simulink model "Demo_CarRealTime2D_cs"  (R2014b)
settings: Solver=ode5  SolverMode=SingleTasking  StartTime=0.0  StopTime=inf  FixedStep=1/1000  RelTol=1e-3
PreLoadFcn:
  | mbxruntime.callbacks.PreLoadFcn(bdroot);
  | check_NUTS_defined;
  | assignin('base',['model_closed_' bdroot],false);
  | addpath('../includes_AEBS');
PostLoadFcn:
  | mbxruntime.callbacks.PostLoadFcn(bdroot);
InitFcn:
  | mbxruntime.callbacks.InitFcn(bdroot);
StartFcn:
  | mbxruntime.callbacks.StartFcn(bdroot);
StopFcn:
  | mbxruntime.callbacks.StopFcn(bdroot);;
  | 
model workspace: external: MAT-File .\Demo_CarRealTime2D_cs_hws.mat (data not in the file)
undefined symbols (not defined in the file or in its folder): Driver_Demands, mbxruntime, tabledata, vicrt_initcallback, vicrt_initmexcallback, vicrt_simulationmanager, warningInitialVelocity, x0
undefined symbols (not defined in the file): Demo_CarRealTime2D_cs_007c1c37f387f47f, Demo_CarRealTime2D_cs_085a64a83ba38cec, Demo_CarRealTime2D_cs_0a7f542d3fc7ab9f, Demo_CarRealTime2D_cs_0d7c72cfaa56dff7, Demo_CarRealTime2D_cs_0de07b35068e3828, Demo_CarRealTime2D_cs_17f4d381375cce95, Demo_CarRealTime2D_cs_1db40a09b08215a9, Demo_CarRealTime2D_cs_2bfa3850c176687b, Demo_CarRealTime2D_cs_35a34f1ba6ce4a22, Demo_CarRealTime2D_cs_378cc77e08d643fb, Demo_CarRealTime2D_cs_409b5c3befba0000, Demo_CarRealTime2D_cs_42628ca5bb62d2f3, Demo_CarRealTime2D_cs_56554a2db408a7f8, Demo_CarRealTime2D_cs_59527455249d7429, Demo_CarRealTime2D_cs_5983ee1b8112afac, Demo_CarRealTime2D_cs_5b5ebcf3ed7bf8e6, Demo_CarRealTime2D_cs_63cbe7fbe16cd5d9, Demo_CarRealTime2D_cs_6e17b9adbf989abf, Demo_CarRealTime2D_cs_6f662a34e5d9a196, Demo_CarRealTime2D_cs_75c4ee8892821e19, Demo_CarRealTime2D_cs_7c64486355814be2, Demo_CarRealTime2D_cs_849809550a2230ef, Demo_CarRealTime2D_cs_87f899bcbe16d8f5, Demo_CarRealTime2D_cs_8e7b50dac25b68a2, Demo_CarRealTime2D_cs_94938e5260f139b3, Demo_CarRealTime2D_cs_983acc940698d1d1, Demo_CarRealTime2D_cs_9d554c72797f76fd, Demo_CarRealTime2D_cs_9d747ee2f15c057f, Demo_CarRealTime2D_cs_ad62a2084d31e898, Demo_CarRealTime2D_cs_b56c8c5f000d30f0, Demo_CarRealTime2D_cs_b95f1b7356e926cc, Demo_CarRealTime2D_cs_BMW_X5_1_Path_pathUniqueID, Demo_CarRealTime2D_cs_BMW_Z3_2_Dynamics_Empty_STATE_BMW_Z3_2_x0, Demo_CarRealTime2D_cs_BMW_Z3_2_Dynamics_Empty_STATE_BMW_Z3_2_y0, Demo_CarRealTime2D_cs_BMW_Z3_2_Dynamics_Empty_STATE_BMW_Z3_2_z0, Demo_CarRealTime2D_cs_BMW_Z3_Path_pathUniqueID, Demo_CarRealTime2D_cs_BMW_Z3_SpeedProfile_speedProfileUniqueID, Demo_CarRealTime2D_cs_c8847ab2e5633224, Demo_CarRealTime2D_cs_c9a0d701286b93fb, Demo_CarRealTime2D_cs_ce758cae7dd1b283, Demo_CarRealTime2D_cs_CrossingPedestrian_Path_pathUniqueID, Demo_CarRealTime2D_cs_CuttingInVehicle_Path_pathUniqueID, Demo_CarRealTime2D_cs_d901ab1c1d2e40bc, Demo_CarRealTime2D_cs_dff70430e5a00a86, Demo_CarRealTime2D_cs_ef038a4f619ad32e, Demo_CarRealTime2D_cs_Female_OverweightAni_1_Path_pathUniqueID, Demo_CarRealTime2D_cs_Ford_Fiesta_1_Path_pathUniqueID, Demo_CarRealTime2D_cs_Ford_FocusWagon_Path_pathUniqueID, Demo_CarRealTime2D_cs_Sphere_1_Dynamics_Empty_STATE_Sphere_1_x0, Demo_CarRealTime2D_cs_Sphere_1_Dynamics_Empty_STATE_Sphere_1_y0, Demo_CarRealTime2D_cs_Sphere_1_Dynamics_Empty_STATE_Sphere_1_z0, WheelL0, WheelL1, WheelR0, WheelR1
libraries: PreScanSimulinkLibrary x15, simulink x15, simulink_extras x15, PreScanUsefulBlocks x2, dspsigops x1
(part 13 of 17)

== system Demo_CarRealTime2D_cs/WheelR1_Ford_FocusWagon/Actuator/visu_Translate ==
  In1 : Inport
  sfun_PositionActuator : S-Function  FunctionName=sfun_PositionActuator  Parameters=SParameter1, SParameter2, SampleTime  EnableBusSupport=off  mask(Legacy Function){SFunctionSpec=void prescan_outputFcn(void ** work1,  PRESCAN_XYZ_DATA u1[1]), SParameter1=uint8([Object3DID 0]), SParameter2=UniqueID, SampleTime=TimeStep, ShowSpec=on}
      mask prompts: SParameter1 "P1:"; SParameter2 "P2:"; SampleTime "Sample time (-1 for inherited):"; ShowSpec "Display function specification"
      mask help:
      | This block allows you to call the legacy functions specified by the following Legacy Code Tool definition:
      | def.SFunctionName = 'sfun_PositionActuator';
      | def.OutputFcnSpec = 'void prescan_outputFcn(void ** work1,  PRESCAN_XYZ_DATA u1[1])';
      | def.StartFcnSpec = 'void prescan_startFcn(void ** work1, uint8 p1[], double p2)';
      | def.TerminateFcnSpec = 'void prescan_terminateFcn(void ** work1)';
      | def.HeaderFiles = {'prescan_positionactuator_data.h', 'prescan_header_data.h', 'prescan_SFunLibrary.h', 'prescan_CreateLogHandler.h', 'prescan_CreateErrorHandler.h'};
      | def.SourceFiles = {'prescan_MexLogHandler.cpp', 'prescan_SimStructErrorHandler.cpp', 'prescan_ConcurrentLogHandler.cpp', 'prescan_ConcurrentErrorHandler.cpp'};
      | def.HostLibFiles = {'sensorinterfaced.lib'};
      | def.TargetLibFiles = {'sensorinterfaced.so'};
      | def.IncPaths = {'.', 'C:\prescandev\vislibrary\vis\..\pimp\include\sensors\InterfaceRTW'};
      | def.SrcPaths = {'.'};
      | def.LibPaths = {'C:\\prescandev\\vislibrary_build\lib'};
      | def.SampleTime = 'parameterized';
      mask Help: <p>This block was generated automatically by the Legacy Code Tool. For detailed help on this tool, call<a href="matlab:legacy_code('help')"> legacy_code('help')</a>.</p>
      mask Callback ShowSpec:
      | if strcmp(get_param(gcbh, 'ShowSpec'), 'on')
      |   set_param(gcbh, 'MaskDisplay', sprintf('fprintf(''%s'');', get_param(gcbh, 'SFunctionSpec')));
      | else
      |   set_param(gcbh, 'MaskDisplay', sprintf('fprintf(''%s'');', get_param(gcbh, 'FunctionName')));
      | end
      mask Display: fprintf('void prescan_outputFcn(void ** work1,  PRESCAN_XYZ_DATA u1[1])');
  wires:
  In1/1 -> sfun_PositionActuator/1

== system Demo_CarRealTime2D_cs/WheelR1_HostVehicle/Actuator/visu_Rotate ==
  In1 : Inport
  sfun_RPYActuator : S-Function  FunctionName=sfun_RPYActuator  Parameters=SParameter1, SParameter2, SampleTime  EnableBusSupport=off  mask(Legacy Function){SFunctionSpec=void prescan_outputFcn(void ** work1,  PRESCAN_XYZ_DATA u1[1]), SParameter1=UniqueID, SParameter2=uint8([Object3DID 0]), SampleTime=TimeStep, ShowSpec=on}
      mask prompts: SParameter1 "P1:"; SParameter2 "P2:"; SampleTime "Sample time (-1 for inherited):"; ShowSpec "Display function specification"
      mask help:
      | This block allows you to call the legacy functions specified by the following Legacy Code Tool definition:
      | def.SFunctionName = 'sfun_PositionActuator';
      | def.OutputFcnSpec = 'void prescan_outputFcn(void ** work1,  PRESCAN_XYZ_DATA u1[1])';
      | def.StartFcnSpec = 'void prescan_startFcn(void ** work1, uint8 p1[], double p2)';
      | def.TerminateFcnSpec = 'void prescan_terminateFcn(void ** work1)';
      | def.HeaderFiles = {'prescan_positionactuator_data.h', 'prescan_header_data.h', 'prescan_SFunLibrary.h', 'prescan_CreateLogHandler.h', 'prescan_CreateErrorHandler.h'};
      | def.SourceFiles = {'prescan_MexLogHandler.cpp', 'prescan_SimStructErrorHandler.cpp', 'prescan_ConcurrentLogHandler.cpp', 'prescan_ConcurrentErrorHandler.cpp'};
      | def.HostLibFiles = {'sensorinterfaced.lib'};
      | def.TargetLibFiles = {'sensorinterfaced.so'};
      | def.IncPaths = {'.', 'C:\prescandev\vislibrary\vis\..\pimp\include\sensors\InterfaceRTW'};
      | def.SrcPaths = {'.'};
      | def.LibPaths = {'C:\\prescandev\\vislibrary_build\lib'};
      | def.SampleTime = 'parameterized';
      mask Help: <p>This block was generated automatically by the Legacy Code Tool. For detailed help on this tool, call<a href="matlab:legacy_code('help')"> legacy_code('help')</a>.</p>
      mask Callback ShowSpec:
      | if strcmp(get_param(gcbh, 'ShowSpec'), 'on')
      |   set_param(gcbh, 'MaskDisplay', sprintf('fprintf(''%s'');', get_param(gcbh, 'SFunctionSpec')));
      | else
      |   set_param(gcbh, 'MaskDisplay', sprintf('fprintf(''%s'');', get_param(gcbh, 'FunctionName')));
      | end
      mask Display: fprintf('void prescan_outputFcn(void ** work1,  PRESCAN_RPY_DATA u1[1])');
  wires:
  In1/1 -> sfun_RPYActuator/1

== system Demo_CarRealTime2D_cs/WheelR1_HostVehicle/Actuator/visu_Translate ==
  In1 : Inport
  sfun_PositionActuator : S-Function  FunctionName=sfun_PositionActuator  Parameters=SParameter1, SParameter2, SampleTime  EnableBusSupport=off  mask(Legacy Function){SFunctionSpec=void prescan_outputFcn(void ** work1,  PRESCAN_XYZ_DATA u1[1]), SParameter1=uint8([Object3DID 0]), SParameter2=UniqueID, SampleTime=TimeStep, ShowSpec=on}
      mask prompts: SParameter1 "P1:"; SParameter2 "P2:"; SampleTime "Sample time (-1 for inherited):"; ShowSpec "Display function specification"
      mask help:
      | This block allows you to call the legacy functions specified by the following Legacy Code Tool definition:
      | def.SFunctionName = 'sfun_PositionActuator';
      | def.OutputFcnSpec = 'void prescan_outputFcn(void ** work1,  PRESCAN_XYZ_DATA u1[1])';
      | def.StartFcnSpec = 'void prescan_startFcn(void ** work1, uint8 p1[], double p2)';
      | def.TerminateFcnSpec = 'void prescan_terminateFcn(void ** work1)';
      | def.HeaderFiles = {'prescan_positionactuator_data.h', 'prescan_header_data.h', 'prescan_SFunLibrary.h', 'prescan_CreateLogHandler.h', 'prescan_CreateErrorHandler.h'};
      | def.SourceFiles = {'prescan_MexLogHandler.cpp', 'prescan_SimStructErrorHandler.cpp', 'prescan_ConcurrentLogHandler.cpp', 'prescan_ConcurrentErrorHandler.cpp'};
      | def.HostLibFiles = {'sensorinterfaced.lib'};
      | def.TargetLibFiles = {'sensorinterfaced.so'};
      | def.IncPaths = {'.', 'C:\prescandev\vislibrary\vis\..\pimp\include\sensors\InterfaceRTW'};
      | def.SrcPaths = {'.'};
      | def.LibPaths = {'C:\\prescandev\\vislibrary_build\lib'};
      | def.SampleTime = 'parameterized';
      mask Help: <p>This block was generated automatically by the Legacy Code Tool. For detailed help on this tool, call<a href="matlab:legacy_code('help')"> legacy_code('help')</a>.</p>
      mask Callback ShowSpec:
      | if strcmp(get_param(gcbh, 'ShowSpec'), 'on')
      |   set_param(gcbh, 'MaskDisplay', sprintf('fprintf(''%s'');', get_param(gcbh, 'SFunctionSpec')));
      | else
      |   set_param(gcbh, 'MaskDisplay', sprintf('fprintf(''%s'');', get_param(gcbh, 'FunctionName')));
      | end
      mask Display: fprintf('void prescan_outputFcn(void ** work1,  PRESCAN_XYZ_DATA u1[1])');
  wires:
  In1/1 -> sfun_PositionActuator/1

== system Demo_CarRealTime2D_cs/Actros_2541_1/SELF_Demux/compas converter/cart2compas ==
  Angle [deg] : Inport
  Constant : Constant  Value=90
  Constant1 : Constant  Value=360
  Gain : Gain  Gain=1/360
  Gain1 : Gain  Gain=360
  Gain2 : Gain  Gain=-1
  Rounding Function : Rounding
  Sum : Sum  Inputs=|-+
  Sum1 : Sum  Inputs=-+|
  Sum2 : Sum  Inputs=++|
  heading [deg] : Outport
  wires:
  Gain/1 -> Rounding Function/1
  Rounding Function/1 -> Gain1/1
  Gain1/1 -> Sum/1
  Angle [deg]/1 -> Sum1/2
  Sum/1 -> Gain2/1
  Sum1/1 -> Gain/1, Sum/2
  Constant/1 -> Sum1/1
  Gain2/1 -> Sum2/2
  Constant1/1 -> Sum2/1
  Sum2/1 -> heading [deg]/1

== system Demo_CarRealTime2D_cs/BMW_X5_1/SELF_Demux/compas converter/cart2compas ==
  Angle [deg] : Inport
  Constant : Constant  Value=90
  Constant1 : Constant  Value=360
  Gain : Gain  Gain=1/360
  Gain1 : Gain  Gain=360
  Gain2 : Gain  Gain=-1
  Rounding Function : Rounding
  Sum : Sum  Inputs=|-+
  Sum1 : Sum  Inputs=-+|
  Sum2 : Sum  Inputs=++|
  heading [deg] : Outport
  wires:
  Gain/1 -> Rounding Function/1
  Rounding Function/1 -> Gain1/1
  Gain1/1 -> Sum/1
  Angle [deg]/1 -> Sum1/2
  Sum/1 -> Gain2/1
  Sum1/1 -> Gain/1, Sum/2
  Constant/1 -> Sum1/1
  Gain2/1 -> Sum2/2
  Constant1/1 -> Sum2/1
  Sum2/1 -> heading [deg]/1

== system Demo_CarRealTime2D_cs/BMW_Z3/SELF_Demux/compas converter/cart2compas ==
  Angle [deg] : Inport
  Constant : Constant  Value=90
  Constant1 : Constant  Value=360
  Gain : Gain  Gain=1/360
  Gain1 : Gain  Gain=360
  Gain2 : Gain  Gain=-1
  Rounding Function : Rounding
  Sum : Sum  Inputs=|-+
  Sum1 : Sum  Inputs=-+|
  Sum2 : Sum  Inputs=++|
  heading [deg] : Outport
  wires:
  Gain/1 -> Rounding Function/1
  Rounding Function/1 -> Gain1/1
  Gain1/1 -> Sum/1
  Angle [deg]/1 -> Sum1/2
  Sum/1 -> Gain2/1
  Sum1/1 -> Gain/1, Sum/2
  Constant/1 -> Sum1/1
  Gain2/1 -> Sum2/2
  Constant1/1 -> Sum2/1
  Sum2/1 -> heading [deg]/1

== system Demo_CarRealTime2D_cs/BMW_Z3_2/SELF_Demux/compas converter/cart2compas ==
  Angle [deg] : Inport
  Constant : Constant  Value=90
  Constant1 : Constant  Value=360
  Gain : Gain  Gain=1/360
  Gain1 : Gain  Gain=360
  Gain2 : Gain  Gain=-1
  Rounding Function : Rounding
  Sum : Sum  Inputs=|-+
  Sum1 : Sum  Inputs=-+|
  Sum2 : Sum  Inputs=++|
  heading [deg] : Outport
  wires:
  Gain/1 -> Rounding Function/1
  Rounding Function/1 -> Gain1/1
  Gain1/1 -> Sum/1
  Angle [deg]/1 -> Sum1/2
  Sum/1 -> Gain2/1
  Sum1/1 -> Gain/1, Sum/2
  Constant/1 -> Sum1/1
  Gain2/1 -> Sum2/2
  Constant1/1 -> Sum2/1
  Sum2/1 -> heading [deg]/1

== system Demo_CarRealTime2D_cs/CrossingPedestrian/SELF_Demux/compas converter/cart2compas ==
  Angle [deg] : Inport
  Constant : Constant  Value=90
  Constant1 : Constant  Value=360
  Gain : Gain  Gain=1/360
  Gain1 : Gain  Gain=360
  Gain2 : Gain  Gain=-1
  Rounding Function : Rounding
  Sum : Sum  Inputs=|-+
  Sum1 : Sum  Inputs=-+|
  Sum2 : Sum  Inputs=++|
  heading [deg] : Outport
  wires:
  Gain/1 -> Rounding Function/1
  Rounding Function/1 -> Gain1/1
  Gain1/1 -> Sum/1
  Angle [deg]/1 -> Sum1/2
  Sum/1 -> Gain2/1
  Sum1/1 -> Gain/1, Sum/2
  Constant/1 -> Sum1/1
  Gain2/1 -> Sum2/2
  Constant1/1 -> Sum2/1
  Sum2/1 -> heading [deg]/1

== system Demo_CarRealTime2D_cs/CuttingInVehicle/SELF_Demux/compas converter/cart2compas ==
  Angle [deg] : Inport
  Constant : Constant  Value=90
  Constant1 : Constant  Value=360
  Gain : Gain  Gain=1/360
  Gain1 : Gain  Gain=360
  Gain2 : Gain  Gain=-1
  Rounding Function : Rounding
  Sum : Sum  Inputs=|-+
  Sum1 : Sum  Inputs=-+|
  Sum2 : Sum  Inputs=++|
  heading [deg] : Outport
  wires:
  Gain/1 -> Rounding Function/1
  Rounding Function/1 -> Gain1/1
  Gain1/1 -> Sum/1
  Angle [deg]/1 -> Sum1/2
  Sum/1 -> Gain2/1
  Sum1/1 -> Gain/1, Sum/2
  Constant/1 -> Sum1/1
  Gain2/1 -> Sum2/2
  Constant1/1 -> Sum2/1
  Sum2/1 -> heading [deg]/1

== system Demo_CarRealTime2D_cs/CuttingInVehicle/Trajectories1/Traj2State1/Traj2State2 ==
  traj : Inport
  MuxState : Subsystem
  Traj2MuxState_Ext : Subsystem
  state : Outport
  wires:
  traj/1 -> Traj2MuxState_Ext/1(Traj)
  MuxState/1(state) -> state/1
  Traj2MuxState_Ext/1(x [m]) -> MuxState/1(x [m])
  Traj2MuxState_Ext/2(y [m]) -> MuxState/2(y [m])
  Traj2MuxState_Ext/3(z [m]) -> MuxState/3(z [m])
  Traj2MuxState_Ext/4(dx [m/s]) -> MuxState/4(dx [m/s])
  Traj2MuxState_Ext/5(dy [m/s]) -> MuxState/5(dy [m/s])
  Traj2MuxState_Ext/6(dz [m/s]) -> MuxState/6(dz [m/s])
  Traj2MuxState_Ext/7(R [rad]) -> MuxState/7(R [rad])
  Traj2MuxState_Ext/8(P [rad]) -> MuxState/8(P [rad])
  Traj2MuxState_Ext/9(Y [rad]) -> MuxState/9(Y [rad])

== system Demo_CarRealTime2D_cs/CuttingInVehicle/Trajectories1/Trajectory_Host_AllSystems/Embeded MATLAB S-Function ==
  gain : Inport
  offset : Inport  Port=2
  MATLAB Function : MATLAB Function  TreatAsAtomicUnit=on  SystemSampleTime=TimeStep
  pos : Outport
  wires:
  offset/1 -> MATLAB Function/2(offset)
  gain/1 -> MATLAB Function/1(gain)
  MATLAB Function/1(y) -> pos/1

== system Demo_CarRealTime2D_cs/Female_OverweightAni_1/SELF_Demux/compas converter/cart2compas ==
  Angle [deg] : Inport
  Constant : Constant  Value=90
  Constant1 : Constant  Value=360
  Gain : Gain  Gain=1/360
  Gain1 : Gain  Gain=360
  Gain2 : Gain  Gain=-1
  Rounding Function : Rounding
  Sum : Sum  Inputs=|-+
  Sum1 : Sum  Inputs=-+|
  Sum2 : Sum  Inputs=++|
  heading [deg] : Outport
  wires:
  Gain/1 -> Rounding Function/1
  Rounding Function/1 -> Gain1/1
  Gain1/1 -> Sum/1
  Angle [deg]/1 -> Sum1/2
  Sum/1 -> Gain2/1
  Sum1/1 -> Gain/1, Sum/2
  Constant/1 -> Sum1/1
  Gain2/1 -> Sum2/2
  Constant1/1 -> Sum2/1
  Sum2/1 -> heading [deg]/1

== system Demo_CarRealTime2D_cs/Ford_Fiesta_1/SELF_Demux/compas converter/cart2compas ==
  Angle [deg] : Inport
  Constant : Constant  Value=90
  Constant1 : Constant  Value=360
  Gain : Gain  Gain=1/360
  Gain1 : Gain  Gain=360
  Gain2 : Gain  Gain=-1
  Rounding Function : Rounding
  Sum : Sum  Inputs=|-+
  Sum1 : Sum  Inputs=-+|
  Sum2 : Sum  Inputs=++|
  heading [deg] : Outport
  wires:
  Gain/1 -> Rounding Function/1
  Rounding Function/1 -> Gain1/1
  Gain1/1 -> Sum/1
  Angle [deg]/1 -> Sum1/2
  Sum/1 -> Gain2/1
  Sum1/1 -> Gain/1, Sum/2
  Constant/1 -> Sum1/1
  Gain2/1 -> Sum2/2
  Constant1/1 -> Sum2/1
  Sum2/1 -> heading [deg]/1

== system Demo_CarRealTime2D_cs/Ford_FocusWagon/SELF_Demux/compas converter/cart2compas ==
  Angle [deg] : Inport
  Constant : Constant  Value=90
  Constant1 : Constant  Value=360
  Gain : Gain  Gain=1/360
  Gain1 : Gain  Gain=360
  Gain2 : Gain  Gain=-1
  Rounding Function : Rounding
  Sum : Sum  Inputs=|-+
  Sum1 : Sum  Inputs=-+|
  Sum2 : Sum  Inputs=++|
  heading [deg] : Outport
  wires:
  Gain/1 -> Rounding Function/1
  Rounding Function/1 -> Gain1/1
  Gain1/1 -> Sum/1
  Angle [deg]/1 -> Sum1/2
  Sum/1 -> Gain2/1
  Sum1/1 -> Gain/1, Sum/2
  Constant/1 -> Sum1/1
  Gain2/1 -> Sum2/2
  Constant1/1 -> Sum2/1
  Sum2/1 -> heading [deg]/1

== system Demo_CarRealTime2D_cs/HostVehicle/Dynamics_UserSpecified/VI-CarRealTime/Input_Bus ==
  Driver_Demands.str_swa : Inport
  Driver_Demands.throttle : Inport  Port=2
  Driver_Demands.brake : Inport  Port=3
  Bus2Map : Subsystem
  Inputs : Subsystem
  VicrtBusAssignment : BusAssignment  AssignedSignals=Driver_Demands.str_swa,Driver_Demands.throttle,Driver_Demands.brake
  vicrt input : Outport
  wires:
  Driver_Demands.brake/1 -> VicrtBusAssignment/4
  Driver_Demands.throttle/1 -> VicrtBusAssignment/3
  Driver_Demands.str_swa/1 -> VicrtBusAssignment/2
  Inputs/1(Inputs) -> VicrtBusAssignment/1  "Inputs"
  VicrtBusAssignment/1 -> Bus2Map/1(Bus In)
  Bus2Map/1(Map Out) -> vicrt input/1

== system Demo_CarRealTime2D_cs/HostVehicle/Dynamics_UserSpecified/VI-CarRealTime/Output_Bus ==
  Outputs : Inport
  IOmap2bus : Subsystem
  VicrtBusSelector : BusSelector  InitFcn=warning('off','Simulink:blocks:BusSelectorDuplicateLeafSignalInMuxedOutput');  StartFcn=warning('on','Simulink:blocks:BusSelectorDuplicateLeafSignalInMuxedOutput');  OutputSignals=ges_chassis_XFORM.X,ges_chassis_XFORM.Y,ges_chassis_XFORM.Z,Vehicle.CM_Body_Fixed_Vx,Vehicle.CM_Body_Fixed_Vy,Vehicle.CM_Body_Fixed_Vz,Vehicle.Euler_Roll,Vehicle.Pitch,Vehicle.Yaw,Wheel.wheel_center_dispz.front_left,Wheel.wheel_center_dispz.front_right,Wheel.wheel_center_dispz.rear_left,Wheel.wheel_center_dispz.rear_right,engine.engine_rpm,Vehicle.CM_Body_Fixed_Ax
  ges_chassis_XFORM.X : Outport
  ges_chassis_XFORM.Y : Outport  Port=2
  ges_chassis_XFORM.Z : Outport  Port=3
  Vehicle.CM_Body_Fixed_Vx : Outport  Port=4
  Vehicle.CM_Body_Fixed_Vy : Outport  Port=5
  Vehicle.CM_Body_Fixed_Vz : Outport  Port=6
  Vehicle.Euler_Roll : Outport  Port=7
  Vehicle.Pitch : Outport  Port=8
  Vehicle.Yaw : Outport  Port=9
  Wheel.wheel_center_dispz.front_left : Outport  Port=10
  Wheel.wheel_center_dispz.front_right : Outport  Port=11
  Wheel.wheel_center_dispz.rear_left : Outport  Port=12
  Wheel.wheel_center_dispz.rear_right : Outport  Port=13
  engine.engine_rpm : Outport  Port=14
  Vehicle.CM_Body_Fixed_Ax : Outport  Port=15
  wires:
  VicrtBusSelector/15 -> Vehicle.CM_Body_Fixed_Ax/1  "<CM_Body_Fixed_Ax>"
  VicrtBusSelector/14 -> engine.engine_rpm/1  "<engine_rpm>"
  VicrtBusSelector/13 -> Wheel.wheel_center_dispz.rear_right/1  "<rear_right>"
  VicrtBusSelector/12 -> Wheel.wheel_center_dispz.rear_left/1  "<rear_left>"
  VicrtBusSelector/11 -> Wheel.wheel_center_dispz.front_right/1  "<front_right>"
  VicrtBusSelector/10 -> Wheel.wheel_center_dispz.front_left/1  "<front_left>"
  VicrtBusSelector/9 -> Vehicle.Yaw/1  "<Yaw>"
  VicrtBusSelector/8 -> Vehicle.Pitch/1  "<Pitch>"
  VicrtBusSelector/7 -> Vehicle.Euler_Roll/1  "<Euler_Roll>"
  VicrtBusSelector/6 -> Vehicle.CM_Body_Fixed_Vz/1  "<CM_Body_Fixed_Vz>"
  VicrtBusSelector/5 -> Vehicle.CM_Body_Fixed_Vy/1  "<CM_Body_Fixed_Vy>"
  VicrtBusSelector/4 -> Vehicle.CM_Body_Fixed_Vx/1  "<CM_Body_Fixed_Vx>"
  VicrtBusSelector/3 -> ges_chassis_XFORM.Z/1  "<Z>"
  VicrtBusSelector/2 -> ges_chassis_XFORM.Y/1  "<Y>"
  VicrtBusSelector/1 -> ges_chassis_XFORM.X/1  "<X>"
  Outputs/1 -> IOmap2bus/1(In)
  IOmap2bus/1(Out) -> VicrtBusSelector/1

== system Demo_CarRealTime2D_cs/HostVehicle/Dynamics_UserSpecified/VI-CarRealTime/vicrt_mex Standard ==
  In1 : Inport
  vicrt_mex : S-Function  InitFcn=vicrt_initmexcallback(gcb);  FunctionName=vicrt_mex  Parameters=vicrt_inputfile,vicrt_outprefix,AniFlag,intStep,inpPortDim,outPortDim  EnableBusSupport=off
  Out1 : Outport
  wires:
  In1/1 -> vicrt_mex/1
  vicrt_mex/1 -> Out1/1

== system Demo_CarRealTime2D_cs/HostVehicle/PathFollower_Preview_1/LateralController/Calculate delta steering error ==
  In1 : Inport
  In2 : Inport  Port=2
  In3 : Inport  Port=3
  In4 : Inport  Port=4
  In5 : Inport  Port=5
  In6 : Inport  Port=6
  In7 : Inport  Port=7
  In8 : Inport  Port=8
  In9 : Inport  Port=9
  In10 : Inport  Port=10
  In11 : Inport  Port=11
  In12 : Inport  Port=12
  eml_delta_steering_error : MATLAB Function  TreatAsAtomicUnit=on  RTWFcnName=sfun_delta_steering_error  RTWFileName=sfun_delta_steering_error
      settings: RTWFileNameOpts=User specified
  Out1 : Outport
  wires:
  In3/1 -> eml_delta_steering_error/3(t_Preview_LatCtrl)
  In2/1 -> eml_delta_steering_error/2(v_x_vehicle_Min)
  In12/1 -> eml_delta_steering_error/12(wheelbase)
  In11/1 -> eml_delta_steering_error/11(Pos_x_CoG_Vehicle)
  In10/1 -> eml_delta_steering_error/10(e_Lat)
  In9/1 -> eml_delta_steering_error/9(inertia_z_vehicle_total)
  In8/1 -> eml_delta_steering_error/8(m_vehicle_total)
  eml_delta_steering_error/1(delta_steeringwheeltotal) -> Out1/1
  In7/1 -> eml_delta_steering_error/7(CorneringStiffness_Tyres_Rear)
  In6/1 -> eml_delta_steering_error/6(CorneringStiffness_Tyres_Front)
  In5/1 -> eml_delta_steering_error/5(yawrate_vehicle)
  In4/1 -> eml_delta_steering_error/4(v_y_vehicle)
  In1/1 -> eml_delta_steering_error/1(v_x_vehicle)

== system Demo_CarRealTime2D_cs/HostVehicle/PathFollower_Preview_1/LateralController/SteeringWheelAngle ==
  Angle_Steering[rad] : Inport
  i_Steering[] : Inport  Port=2
  Angle_SteeringWheel_Last[deg] : Inport  Port=3
  LatCtrl1_Enable[0Off|1On] : Inport  Port=4
  Angle_Max_SteeringWheel[deg]1 : Constant  Value=Angle_Max_SteeringWheel  SampleTime=CSSampleTime
  Const_t_PT1_LatCtrl[s] : Constant  Value=DelayTime  SampleTime=CSSampleTime
  FirstOrderDynamics : Subsystem  mask(First Order Dynamics){}
      mask Display:
      | port_label('input',1,'In')
      | port_label('input',2,'T')
      | port_label('input',3,'Reset')
      | port_label('input',4,'x0')
      | 
      | plot([0.4 0.95], [0.1 0.1]);
      | plot([0.4 0.4], [0.1 0.95]);
      | plot(0.4 + 0.5*[0:0.1:1],0.8- 0.7 * exp(-5*[0:0.1:1]));
  Gain : Gain  SaturateOnIntegerOverflow=on  OutDataTypeStr=Inherit: Same as input  ParamDataTypeStr=Inherit: Same as input
  Product : Product  SaturateOnIntegerOverflow=on  OutDataTypeStr=Inherit: Same as first input
  Rate Limiter : RateLimiter  RisingSlewLimit=MaxSteeringRate  FallingSlewLimit=-MaxSteeringRate  SampleTimeMode=inherited
  Sat_Total : Subsystem
      mask Display:
      | plot([0.25 0.4 0.6 0.75],[0.2 0.2 0.8 0.8])
      | port_label('input',2,'Lim')
      | port_label('output',2,'Info')
  Terminator1 : Terminator
  rad2deg : Gain  Gain=180/pi  SaturateOnIntegerOverflow=on  OutDataTypeStr=Inherit: Same as input  ParamDataTypeStr=Inherit: Same as input
  Angle_SteeringWheel[deg] : Outport
  wires:
  Rate Limiter/1 -> FirstOrderDynamics/1(In)
  Gain/1 -> FirstOrderDynamics/3(Reset)
  Angle_SteeringWheel_Last[deg]/1 -> FirstOrderDynamics/4(x0)
  LatCtrl1_Enable[0Off|1On]/1 -> Gain/1
  Const_t_PT1_LatCtrl[s]/1 -> FirstOrderDynamics/2(TimeConstant[s])
  Sat_Total/2(Sat_Info) -> Terminator1/1
  Angle_Steering[rad]/1 -> rad2deg/1
  i_Steering[]/1 -> Product/2
  rad2deg/1 -> Product/1
  Product/1 -> Sat_Total/1(In)
  Sat_Total/1(Sat_Total) -> Rate Limiter/1
  FirstOrderDynamics/1(Out) -> Angle_SteeringWheel[deg]/1
  Angle_Max_SteeringWheel[deg]1/1 -> Sat_Total/2(Sat_Limit)

== system Demo_CarRealTime2D_cs/HostVehicle/PathFollower_Preview_1/LateralController/s_Preview_LatCtrl ==
  v_x_Vehicle[m|s] : Inport
  v_x_Vehicle_Min[m|s] : Inport  Port=2
  t_Preview_LatCtrl[s] : Inport  Port=3
  Max : MinMax  Function=max  Inputs=2  SaturateOnIntegerOverflow=on  InputSameDT=on
  Prod_s_Min : Product  SaturateOnIntegerOverflow=on  OutDataTypeStr=Inherit: Same as first input
  Product : Product  SaturateOnIntegerOverflow=on  OutDataTypeStr=Inherit: Same as first input
  s_Preview_LatCtrl[m] : Outport
  wires:
  Max/1 -> s_Preview_LatCtrl[m]/1
  Prod_s_Min/1 -> Max/2
  v_x_Vehicle_Min[m|s]/1 -> Prod_s_Min/2
  t_Preview_LatCtrl[s]/1 -> Prod_s_Min/1, Product/2
  Product/1 -> Max/1
  v_x_Vehicle[m|s]/1 -> Product/1

== system Demo_CarRealTime2D_cs/HostVehicle/PathFollower_Preview_1/LongitudinalController/Check_Initial_Velocity ==
  " v_actual_[m|s]" : Inport
  Initial_Velocity_[m|s] : Inport  Port=2
  > eps : simulink/Logic and Bit Operations/Compare To Constant  relop=>  const=0.1  OutDataTypeStr=boolean
  Abs : Abs
  Assertion : Assertion  AssertionFailFcn=warningInitialVelocity(PathFollowerBlockPath);  StopWhenAssertionFail=off
  Constant : Constant  Value=false
  First ? : Memory  X0=1
  Logical Operator : Logic  AllPortsSameDT=off  OutDataTypeStr=boolean
  Logical Operator1 : Logic  Operator=NOT  AllPortsSameDT=off  OutDataTypeStr=boolean
  Sum : Sum  Inputs=+-
  wires:
  Logical Operator1/1 -> Assertion/1
  Logical Operator/1 -> Logical Operator1/1
  Constant/1 -> First ?/1
  First ?/1 -> Logical Operator/2
  > eps/1 -> Logical Operator/1
  Sum/1 -> Abs/1
  Abs/1 -> > eps/1
  Initial_Velocity_[m|s]/1 -> Sum/2
  " v_actual_[m|s]"/1 -> Sum/1

== system Demo_CarRealTime2D_cs/HostVehicle/PathFollower_Preview_1/LongitudinalController/If Desired Velocity = 0 ==
  In1 : Inport
  Action Port : ActionPort  InitializeStates=reset  PropagateVarSize=During execution
  constant : Constant  Value=0
  constant1 : Constant  Value=150
  throttle [%] : Outport  InitialOutput=[0]
  brake pressure [bar] : Outport  Port=2  InitialOutput=[150]
  Auto_GearShift : Outport  Port=3
  wires:
  In1/1 -> Auto_GearShift/1
  constant/1 -> throttle [%]/1
  constant1/1 -> brake pressure [bar]/1

== system Demo_CarRealTime2D_cs/HostVehicle/PathFollower_Preview_1/LongitudinalController/If Desired Velocity ~= 0 ==
  note: No brake/throttle actions
      | in case of small ctrl error,
      |  in order to prevent nervous
      | ctrl behaviour
  note: CONSTANT VELOCITY CONTROL
  In1 : Inport
  Desired Velocity [m/s] : Inport  Port=2
  Action Port : ActionPort  InitializeStates=reset  PropagateVarSize=During execution
  Dead Zone1 : DeadZone  LowerValue=-10  UpperValue=1  SaturateOnIntegerOverflow=on
  Gain1 : Gain  Gain=-1
  Gain2 : Gain  Gain=1.5
  Limiter_brake : Saturate  UpperLimit=150  LowerLimit=0
  Limiter_throttle : Saturate  UpperLimit=100  LowerLimit=0
  PID_AWU : Subsystem  mask(PID Controller){P=LongCtrl_P, I=LongCtrl_I, D=LongCtrl_D}
      mask prompts: P "Proportional:"; I "Integral:"; D "Derivative:"
      mask help:
      | Enter expressions for proportional, integral, and derivative terms.
      | P+I/s+Ds
      mask Help: This block implements a PID controller where parameters are entered for the Proportional, Integral and Derivative terms. Unmask this block to see how it works. The derivative term is implemented using a true derivative block.
      mask Display: disp('PID')
  throttle [%] : Outport
  brake pressure [bar] : Outport  Port=2
  Auto_GearShift : Outport  Port=3
  wires:
  Dead Zone1/1 -> Gain2/1, Limiter_throttle/1
  Gain1/1 -> Limiter_brake/1
  Gain2/1 -> Gain1/1
  PID_AWU/1(u) -> Dead Zone1/1
  Desired Velocity [m/s]/1 -> PID_AWU/1(e)
  In1/1 -> Auto_GearShift/1
  Limiter_brake/1 -> brake pressure [bar]/1
  Limiter_throttle/1 -> throttle [%]/1  "throttle"

== system Demo_CarRealTime2D_cs/HostVehicle/PathFollower_Preview_1/LongitudinalController/Memory External IC ==
  note: Xnew
  note: Initial Value
  u : Inport
  IC : Inport  Port=2
  FixPt Constant : Constant  DisableCoverage=on  Value=0  OutDataTypeStr=fixdt(0,8,0)
  FixPt Data Type Duplicate1 : DataTypeDuplicate  DisableCoverage=on  NumInputPorts=3
  Init : Switch  Criteria=u2 ~= 0  OutDataTypeStr=Inherit: Inherit via back propagation  ZeroCross=off
  Memory : Memory  X0=1  InheritSampleTime=on
  Memory1 : Memory  InheritSampleTime=on
  y : Outport
  wires:
  Memory1/1 -> Init/3  "Xold"
  Init/1 -> y/1, FixPt Data Type Duplicate1/1
  Memory/1 -> Init/2
  FixPt Constant/1 -> Memory/1
  u/1 -> Memory1/1, FixPt Data Type Duplicate1/2
  IC/1 -> Init/1, FixPt Data Type Duplicate1/3

== system Demo_CarRealTime2D_cs/HostVehicle/SELF_Demux/compas converter/cart2compas ==
  Angle [deg] : Inport
  Constant : Constant  Value=90
  Constant1 : Constant  Value=360
  Gain : Gain  Gain=1/360
  Gain1 : Gain  Gain=360
  Gain2 : Gain  Gain=-1
  Rounding Function : Rounding
  Sum : Sum  Inputs=|-+
  Sum1 : Sum  Inputs=-+|
  Sum2 : Sum  Inputs=++|
  heading [deg] : Outport
  wires:
  Gain/1 -> Rounding Function/1
  Rounding Function/1 -> Gain1/1
  Gain1/1 -> Sum/1
  Angle [deg]/1 -> Sum1/2
  Sum/1 -> Gain2/1
  Sum1/1 -> Gain/1, Sum/2
  Constant/1 -> Sum1/1
  Gain2/1 -> Sum2/2
  Constant1/1 -> Sum2/1
  Sum2/1 -> heading [deg]/1

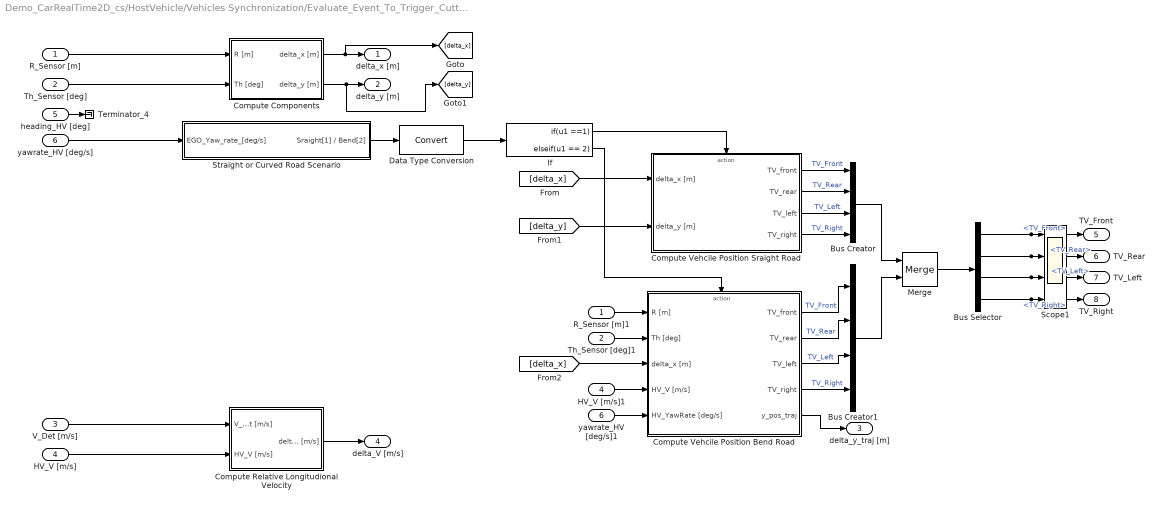
== system Demo_CarRealTime2D_cs/HostVehicle/Vehicles Synchronization/Evaluate_Event_To_Trigger_CuttingVehicle/Evaluate Experiment Conditions  ==
  R_Sensor [m] : Inport
  Th_Sensor [deg] : Inport  Port=2
  V_Det [m/s] : Inport  Port=3
  HV_V [m/s] : Inport  Port=4
  heading_HV [deg] : Inport  Port=5
  yawrate_HV [deg/s] : Inport  Port=6
  Bus Creator : BusCreator
  Bus Creator1 : BusCreator
  Bus Selector : BusSelector  OutputSignals=TV_Front,TV_Rear,TV_Left,TV_Right
  Compute Components : Subsystem
  Compute Relative Longitudional Velocity : Subsystem
  Compute Vehcile Position Bend Road : Subsystem  TreatAsAtomicUnit=on
  Compute Vehcile Position Sraight Road : Subsystem  TreatAsAtomicUnit=on
  Data Type Conversion : DataTypeConversion
  HV_V [m/s]1 : InportShadow  Port=4
  If : If  IfExpression=u1 ==1  ElseIfExpressions=u1 == 2  ShowElse=off
  Merge : Merge
  R_Sensor [m]1 : InportShadow
  Scope1 : Scope  NumInputPorts=4
      settings: YMin=1~0~0~0.95  YMax=2~1~1~1.05
  Straight or Curved Road Scenario : Subsystem
  Terminator_4 : Terminator
  Th_Sensor [deg]1 : InportShadow  Port=2
  yawrate_HV [deg/s]1 : InportShadow  Port=6
  delta_x [m] : Outport
  delta_y [m] : Outport  Port=2
  delta_y_traj [m] : Outport  Port=3
  delta_V [m/s] : Outport  Port=4
  TV_Front : Outport  Port=5
  TV_Rear : Outport  Port=6
  TV_Left : Outport  Port=7
  TV_Right : Outport  Port=8
  wires:
  Bus Selector/4 -> TV_Right/1, Scope1/4  "<TV_Right>"
  Bus Selector/3 -> TV_Left/1, Scope1/3  "<TV_Left>"
  Bus Selector/2 -> TV_Rear/1, Scope1/2  "<TV_Rear>"
  Bus Selector/1 -> TV_Front/1, Scope1/1  "<TV_Front>"
  Compute Vehcile Position Bend Road/5(y_pos_traj) -> delta_y_traj [m]/1
  heading_HV [deg]/1 -> Terminator_4/1
  Merge/1 -> Bus Selector/1
  Bus Creator1/1 -> Merge/2
  Bus Creator/1 -> Merge/1
  Compute Vehcile Position Bend Road/4(TV_right) -> Bus Creator1/4  "TV_Right"
  Compute Vehcile Position Bend Road/3(TV_left) -> Bus Creator1/3  "TV_Left"
  Compute Vehcile Position Bend Road/2(TV_rear) -> Bus Creator1/2  "TV_Rear"
  Compute Vehcile Position Bend Road/1("TV_front ") -> Bus Creator1/1  "TV_Front"
  Compute Vehcile Position Sraight Road/2(TV_rear) -> Bus Creator/2  "TV_Rear"
  Compute Vehcile Position Sraight Road/3(TV_left) -> Bus Creator/3  "TV_Left"
  Compute Vehcile Position Sraight Road/1("TV_front ") -> Bus Creator/1  "TV_Front"
  Compute Vehcile Position Sraight Road/4(TV_right) -> Bus Creator/4  "TV_Right"
  yawrate_HV [deg/s]1/1 -> Compute Vehcile Position Bend Road/5(HV_YawRate [deg/s])
  HV_V [m/s]1/1 -> Compute Vehcile Position Bend Road/4(HV_V [m/s])
  [delta_x] -> Compute Vehcile Position Bend Road/3(delta_x [m])
  [delta_y] -> Compute Vehcile Position Sraight Road/2(delta_y [m])
  [delta_x] -> Compute Vehcile Position Sraight Road/1(delta_x [m])
  Th_Sensor [deg]1/1 -> Compute Vehcile Position Bend Road/2(Th [deg])
  R_Sensor [m]1/1 -> Compute Vehcile Position Bend Road/1(R [m])
  If/2 -> Compute Vehcile Position Bend Road/Action
  If/1 -> Compute Vehcile Position Sraight Road/Action
  Data Type Conversion/1 -> If/1
  Straight or Curved Road Scenario/1(Sraight[1] / Bend[2]) -> Data Type Conversion/1
  yawrate_HV [deg/s]/1 -> Straight or Curved Road Scenario/1(EGO_Yaw_rate_[deg/s])
  Th_Sensor [deg]/1 -> Compute Components/2(Th [deg])
  Compute Relative Longitudional Velocity/1(delta_V [m/s]) -> delta_V [m/s]/1
  HV_V [m/s]/1 -> Compute Relative Longitudional Velocity/2(HV_V [m/s])
  V_Det [m/s]/1 -> Compute Relative Longitudional Velocity/1(V_Det [m/s])
  Compute Components/2(delta_y [m]) -> [delta_y], delta_y [m]/1
  Compute Components/1(delta_x [m]) -> [delta_x], delta_x [m]/1
  R_Sensor [m]/1 -> Compute Components/1(R [m])

== system Demo_CarRealTime2D_cs/Male_Regular_LeaningBack_2/SELF_Demux/compas converter/cart2compas ==
  Angle [deg] : Inport
  Constant : Constant  Value=90
  Constant1 : Constant  Value=360
  Gain : Gain  Gain=1/360
  Gain1 : Gain  Gain=360
  Gain2 : Gain  Gain=-1
  Rounding Function : Rounding
  Sum : Sum  Inputs=|-+
  Sum1 : Sum  Inputs=-+|
  Sum2 : Sum  Inputs=++|
  heading [deg] : Outport
  wires:
  Gain/1 -> Rounding Function/1
  Rounding Function/1 -> Gain1/1
  Gain1/1 -> Sum/1
  Angle [deg]/1 -> Sum1/2
  Sum/1 -> Gain2/1
  Sum1/1 -> Gain/1, Sum/2
  Constant/1 -> Sum1/1
  Gain2/1 -> Sum2/2
  Constant1/1 -> Sum2/1
  Sum2/1 -> heading [deg]/1

== system Demo_CarRealTime2D_cs/Sphere_1/SELF_Demux/compas converter/cart2compas ==
  Angle [deg] : Inport
  Constant : Constant  Value=90
  Constant1 : Constant  Value=360
  Gain : Gain  Gain=1/360
  Gain1 : Gain  Gain=360
  Gain2 : Gain  Gain=-1
  Rounding Function : Rounding
  Sum : Sum  Inputs=|-+
  Sum1 : Sum  Inputs=-+|
  Sum2 : Sum  Inputs=++|
  heading [deg] : Outport
  wires:
  Gain/1 -> Rounding Function/1
  Rounding Function/1 -> Gain1/1
  Gain1/1 -> Sum/1
  Angle [deg]/1 -> Sum1/2
  Sum/1 -> Gain2/1
  Sum1/1 -> Gain/1, Sum/2
  Constant/1 -> Sum1/1
  Gain2/1 -> Sum2/2
  Constant1/1 -> Sum2/1
  Sum2/1 -> heading [deg]/1

== system Demo_CarRealTime2D_cs/Toyota_Previa_1/SELF_Demux/compas converter/cart2compas ==
  Angle [deg] : Inport
  Constant : Constant  Value=90
  Constant1 : Constant  Value=360
  Gain : Gain  Gain=1/360
  Gain1 : Gain  Gain=360
  Gain2 : Gain  Gain=-1
  Rounding Function : Rounding
  Sum : Sum  Inputs=|-+
  Sum1 : Sum  Inputs=-+|
  Sum2 : Sum  Inputs=++|
  heading [deg] : Outport
  wires:
  Gain/1 -> Rounding Function/1
  Rounding Function/1 -> Gain1/1
  Gain1/1 -> Sum/1
  Angle [deg]/1 -> Sum1/2
  Sum/1 -> Gain2/1
  Sum1/1 -> Gain/1, Sum/2
  Constant/1 -> Sum1/1
  Gain2/1 -> Sum2/2
  Constant1/1 -> Sum2/1
  Sum2/1 -> heading [deg]/1

== system Demo_CarRealTime2D_cs/CuttingInVehicle/Trajectories1/Traj2State1/Traj2State2/MuxState ==
  x [m] : Inport
  y [m] : Inport  Port=2
  z [m] : Inport  Port=3
  dx [m/s] : Inport  Port=4
  dy [m/s] : Inport  Port=5
  dz [m/s] : Inport  Port=6
  R [rad] : Inport  Port=7
  P [rad] : Inport  Port=8
  Y [rad] : Inport  Port=9
  Mux : Mux  Inputs=9
  state : Outport
  wires:
  Mux/1 -> state/1
  dx [m/s]/1 -> Mux/4
  dy [m/s]/1 -> Mux/5
  dz [m/s]/1 -> Mux/6
  R [rad]/1 -> Mux/7
  P [rad]/1 -> Mux/8
  Y [rad]/1 -> Mux/9
  x [m]/1 -> Mux/1
  y [m]/1 -> Mux/2
  z [m]/1 -> Mux/3

== system Demo_CarRealTime2D_cs/CuttingInVehicle/Trajectories1/Traj2State1/Traj2State2/Traj2MuxState_Ext ==
  Traj : Inport
  Terminator{1..9} (9 alike) : Terminator
  demux : Subsystem
  x [m] : Outport
  y [m] : Outport  Port=2
  z [m] : Outport  Port=3
  dx [m/s] : Outport  Port=4
  dy [m/s] : Outport  Port=5
  dz [m/s] : Outport  Port=6
  R [rad] : Outport  Port=7
  P [rad] : Outport  Port=8
  Y [rad] : Outport  Port=9
  wires:
  demux/8(P) -> P [rad]/1
  demux/2(y) -> y [m]/1
  demux/1(x) -> x [m]/1
  demux/6(velz) -> dz [m/s]/1
  Traj/1 -> demux/1(traj)
  demux/3(z) -> z [m]/1
  demux/17(accP) -> Terminator6/1
  demux/16(accR) -> Terminator3/1
  demux/18(accY) -> Terminator2/1
  demux/15(accz) -> Terminator7/1
  demux/14(accy) -> Terminator9/1
  demux/13(accx) -> Terminator8/1
  demux/12(velY) -> Terminator1/1
  demux/11(velP) -> Terminator5/1
  demux/10(velR) -> Terminator4/1
  demux/4(velx) -> dx [m/s]/1
  demux/5(vely) -> dy [m/s]/1
  demux/7(R) -> R [rad]/1
  demux/9(Y) -> Y [rad]/1
